simulink library "AEMS_Standard_Library"  (R2016b)
settings: Solver=ode45  StartTime=0.0  StopTime=10.0  RelTol=1e-3
undefined symbols (not defined in the file or in its folder): BkPY, carto, Cbx_extegr, Cbx_lpegrsys, Cbx_portegr, Cnx_bnk_nr_conf, Cnx_cyl_nr_conf, ConfigManagement, configuration_management, Cxx_dcm_io_tmr_end_xxxx, Cxx_dcm_rt_tmr_end, Cxx_DID_xxxx_IO_max, Cxx_DID_xxxx_IO_min, Cxx_egrhsofs, Cxx_vmaniegi, DEM_DEBOUNCE_FREEZE, DEM_DTR_CTL_INVISIBLE, DEM_DTR_CTL_NORMAL, Dem_DtrId2_XXX, Dem_DtrId3_XXX, Dem_DtrId4_XXX, Dem_DtrId5_XXX, Dem_DtrId6_XXX, Dem_DtrId7_XXX, Dem_DtrId8_XXX, Dem_DtrId9_XXX, Dem_DtrId_XXX, Dem_EnableConditionId2_XXX, Dem_EnableConditionId3_XXX, Dem_EnableConditionId4_XXX, Dem_EnableConditionId5_XXX, Dem_EnableConditionId6_XXX, Dem_EnableConditionId7_XXX, Dem_EnableConditionId8_XXX, Dem_EnableConditionId_XXX, Dem_EventId, Dem_EventId2_XXX, Dem_EventId3_XXX, Dem_EventId4_XXX, Dem_EventId5_XXX, Dem_EventId6_XXX, Dem_EventId7_XXX, Dem_EventId8_XXX, Dem_EventId9_XXX, Dem_EventId_Device_Faulttype, Dem_EventId_XXX, DEM_IUMPR_GENERAL_DENOMINATOR, DEM_OPCYC_IGNITION, Dem_RatioId2_XXX, Dem_RatioId3_XXX, Dem_RatioId4_XXX, Dem_RatioId5_XXX, Dem_RatioId6_XXX, Dem_RatioId7_XXX, Dem_RatioId8_XXX, Dem_RatioId_XXX, Dem_StorageConditionId2_XXX, Dem_StorageConditionId3_XXX, Dem_StorageConditionId4_XXX, Dem_StorageConditionId5_XXX ... (+65)
libraries: AEMS_Standard_Library x477, simulink x2
(part 28 of 39)

== system AEMS_Standard_Library/SPECIFIC/AEMS_AT_EHR/A_Enabled_Calculation ==
  Vxx_ehr_sel_tenv : Inport
  Vxx_ehr_cnvt_fac : Inport  Port=2
  Vxx_ehr_ext_exch_ar : Inport  Port=3
  Vxx_ehr_samp_t : Inport  Port=4
  Vxx_ehr_sys_egaf : Inport  Port=5
  Vxx_ehr_wht : Inport  Port=6
  Vxx_ehr_utp : Inport  Port=7
  Vxx_ehr_cata_temp_dly : Inport  Port=8
  Vxx_ehr_exo_pow : Inport  Port=9
  Vxx_ehr_spc_ex_gas_temp_cpy : Inport  Port=10
  Vxx_ehr_spc_cata_temp_cpy : Inport  Port=11
  A_Calcul_for_all_bricks : Subsystem
  B_Temp_calculation_in_brick : Subsystem
  Saturation : Saturate  UpperLimit=65.535  LowerLimit=0  RndMeth=Zero
      settings: AttributesFormatString=<limits=%<UpperLimit>/%<LowerLimit>>
  Vxx_ehr_dtp : Outport
  Vxx_ehr_ext_pow_loss : Outport  Port=2
  Vxx_ehr_wht_entr : Outport  Port=3
  Vxx_ehr_ex_gas_entr : Outport  Port=4
  Vxx_ehr_ext_cnvt_entr : Outport  Port=5
  Vxx_ehr_exo_temp_flu : Outport  Port=6
  Vxx_ehr_wht_temp_flu : Outport  Port=7
  Vxx_ehr_ex_gas_temp_flu : Outport  Port=8
  Vxx_ehr_ext_cnvt_temp_flu : Outport  Port=9
  wires:
  Saturation/1 -> Vxx_ehr_ext_cnvt_entr/1, B_Temp_calculation_in_brick/1(Vxx_ehr_ext_cnvt_entr)
  A_Calcul_for_all_bricks/1(Vxx_ehr_ext_cnvt_entr) -> Saturation/1
  B_Temp_calculation_in_brick/1(Vxx_ehr_dtp) -> Vxx_ehr_dtp/1
  B_Temp_calculation_in_brick/3(Vxx_ehr_wht_entr) -> Vxx_ehr_wht_entr/1
  B_Temp_calculation_in_brick/2(Vxx_ehr_ext_pow_loss) -> Vxx_ehr_ext_pow_loss/1
  Vxx_ehr_sel_tenv/1 -> B_Temp_calculation_in_brick/3(Vxx_ehr_sel_tenv)
  Vxx_ehr_cnvt_fac/1 -> A_Calcul_for_all_bricks/1(Vxx_ehr_cnvt_fac)
  Vxx_ehr_ext_exch_ar/1 -> A_Calcul_for_all_bricks/2(Vxx_ehr_ext_exch_ar)
  Vxx_ehr_samp_t/1 -> A_Calcul_for_all_bricks/3(Vxx_ehr_samp_t), B_Temp_calculation_in_brick/2(Vxx_ehr_samp_t)
  Vxx_ehr_spc_ex_gas_temp_cpy/1 -> B_Temp_calculation_in_brick/4(Vxx_ehr_spc_ex_gas_temp_cpy)
  Vxx_ehr_spc_cata_temp_cpy/1 -> B_Temp_calculation_in_brick/5(Vxx_ehr_spc_cata_temp_cpy)
  Vxx_ehr_sys_egaf/1 -> B_Temp_calculation_in_brick/6(Vxx_ehr_sys_egaf)
  Vxx_ehr_exo_pow/1 -> B_Temp_calculation_in_brick/7(Vxx_ehr_exo_pow)
  Vxx_ehr_wht/1 -> B_Temp_calculation_in_brick/8(Vxx_ehr_wht)
  Vxx_ehr_utp/1 -> B_Temp_calculation_in_brick/9(Vxx_ehr_utp)
  Vxx_ehr_cata_temp_dly/1 -> B_Temp_calculation_in_brick/10(Vxx_ehr_cata_temp_dly)
  B_Temp_calculation_in_brick/8(Vxx_ehr_ext_cnvt_temp_flu) -> Vxx_ehr_ext_cnvt_temp_flu/1
  B_Temp_calculation_in_brick/4(Vxx_ehr_ex_gas_entr) -> Vxx_ehr_ex_gas_entr/1
  B_Temp_calculation_in_brick/5(Vxx_ehr_exo_temp_flu) -> Vxx_ehr_exo_temp_flu/1
  B_Temp_calculation_in_brick/6(Vxx_ehr_wht_temp_flu) -> Vxx_ehr_wht_temp_flu/1
  B_Temp_calculation_in_brick/7(Vxx_ehr_ex_gas_temp_flu) -> Vxx_ehr_ex_gas_temp_flu/1

== system AEMS_Standard_Library/SPECIFIC/AEMS_AT_TUBE/A_Thermal_Calculation ==
  Vxx_tub_utp : Inport
  Vxx_tub_utp_dly : Inport  Port=2
  Vxx_tub_egaf : Inport  Port=3
  Vxx_tub_temp_air : Inport  Port=4
  Vxx_tub_pow_ext : Inport  Port=5
  Vxx_tub_itl_ar : Inport  Port=6
  Vxx_tub_itl_cnvt_fac : Inport  Port=7
  Vxx_tub_ext_ar : Inport  Port=8
  Vxx_tub_ext_cnvt_fac : Inport  Port=9
  Vxx_tub_wht : Inport  Port=10
  Vxx_tub_temp_rd_loss : Inport  Port=11
  Vxx_tub_itl_gas_wht_cor : Inport  Port=12
  Vxx_tub_cal_cpy : Inport  Port=13
  Vxx_tub_gas_cal_cpy : Inport  Port=14
  Vxx_tub_utp_gas_wht_cor : Inport  Port=15
  Vxx_tub_samp_t : Inport  Port=16
  Vxx_tub_temp_esti_dly : Inport  Port=17
  Vxx_tub_ex_gas_dtp_esti_dly : Inport  Port=18
  A_Thermal_Convection_Terms_Tube : Subsystem
  B_Thermal_Material_Model_Tube : Subsystem
  C_Thermal_Gas_Model_Tube : Subsystem
  Saturation : Saturate  UpperLimit=13106  LowerLimit=0  RndMeth=Zero
      settings: AttributesFormatString=<limits=%<UpperLimit>/%<LowerLimit>>
  Saturation1 : Saturate  UpperLimit=65.535  LowerLimit=0  RndMeth=Zero
      settings: AttributesFormatString=<limits=%<UpperLimit>/%<LowerLimit>>
  Saturation2 : Saturate  UpperLimit=32767  LowerLimit=-32767  RndMeth=Zero
      settings: AttributesFormatString=<limits=%<UpperLimit>/%<LowerLimit>>
  Saturation3 : Saturate  UpperLimit=32767  LowerLimit=-32767  RndMeth=Zero
      settings: AttributesFormatString=<limits=%<UpperLimit>/%<LowerLimit>>
  Vxx_tub_ex_gas_dtp_esti : Outport
  Vxx_tub_temp_esti : Outport  Port=2
  Vxx_tub_ex_gas_pow_loss : Outport  Port=3
  Vxx_tub_temp_pow_loss : Outport  Port=4
  Vxx_tub_temp_rd_entr : Outport  Port=5
  Vxx_tub_wht_entr : Outport  Port=6
  Vxx_tub_itl_cnvt_entr : Outport  Port=7
  Vxx_tub_ext_cnvt_entr : Outport  Port=8
  Vxx_tub_entr_tot : Outport  Port=9
  Vxx_tub_ext_cnvt_temp_flu : Outport  Port=10
  Vxx_tub_itl_cnvt_temp_flu : Outport  Port=11
  Vxx_tub_wht_temp_flu : Outport  Port=12
  Vxx_tub_ex_gas_entr : Outport  Port=13
  Vxx_tub_itl_gas_wht_entr : Outport  Port=14
  Vxx_tub_itl_gas_cnvt_entr : Outport  Port=15
  Vxx_tub_gas_entr_tot : Outport  Port=16
  Vxx_tub_gas_temp_flu : Outport  Port=17
  Vxx_tub_gas_wht_temp_flu : Outport  Port=18
  Vxx_tub_gas_itl_cnvt_temp_flu : Outport  Port=19
  Vxx_tub_gas_utp_wht_temp_flu : Outport  Port=20
  Vxx_tub_gas_ext_egy_temp_flu : Outport  Port=21
  wires:
  Saturation3/1 -> Vxx_tub_ex_gas_pow_loss/1
  Saturation2/1 -> Vxx_tub_temp_pow_loss/1
  A_Thermal_Convection_Terms_Tube/1(Vxx_tub_ext_ar_cnvt_fac) -> Saturation1/1
  C_Thermal_Gas_Model_Tube/11(Vxx_tub_gas_ext_egy_temp_flu) -> Vxx_tub_gas_ext_egy_temp_flu/1
  C_Thermal_Gas_Model_Tube/10(Vxx_tub_gas_utp_wht_temp_flu) -> Vxx_tub_gas_utp_wht_temp_flu/1
  C_Thermal_Gas_Model_Tube/9(Vxx_tub_gas_itl_cnvt_temp_flu) -> Vxx_tub_gas_itl_cnvt_temp_flu/1
  C_Thermal_Gas_Model_Tube/8(Vxx_tub_gas_wht_temp_flu) -> Vxx_tub_gas_wht_temp_flu/1
  C_Thermal_Gas_Model_Tube/7(Vxx_tub_gas_temp_flu) -> Vxx_tub_gas_temp_flu/1
  C_Thermal_Gas_Model_Tube/6(Vxx_tub_gas_entr_tot) -> Vxx_tub_gas_entr_tot/1
  C_Thermal_Gas_Model_Tube/5(Vxx_tub_itl_gas_cnvt_entr) -> Vxx_tub_itl_gas_cnvt_entr/1
  C_Thermal_Gas_Model_Tube/4(Vxx_tub_itl_gas_wht_entr) -> Vxx_tub_itl_gas_wht_entr/1
  C_Thermal_Gas_Model_Tube/3(Vxx_tub_ex_gas_entr) -> Vxx_tub_ex_gas_entr/1
  B_Thermal_Material_Model_Tube/10(Vxx_tub_wht_temp_flu) -> Vxx_tub_wht_temp_flu/1
  B_Thermal_Material_Model_Tube/9(Vxx_tub_itl_cnvt_temp_flu) -> Vxx_tub_itl_cnvt_temp_flu/1
  B_Thermal_Material_Model_Tube/8(Vxx_tub_ext_cnvt_temp_flu) -> Vxx_tub_ext_cnvt_temp_flu/1
  B_Thermal_Material_Model_Tube/7(Vxx_tub_entr_tot) -> Vxx_tub_entr_tot/1
  B_Thermal_Material_Model_Tube/6(Vxx_tub_ext_cnvt_entr) -> Vxx_tub_ext_cnvt_entr/1
  B_Thermal_Material_Model_Tube/5(Vxx_tub_itl_cnvt_entr) -> Vxx_tub_itl_cnvt_entr/1
  B_Thermal_Material_Model_Tube/4(Vxx_tub_wht_entr) -> Vxx_tub_wht_entr/1
  B_Thermal_Material_Model_Tube/3(Vxx_tub_temp_rd_entr) -> Vxx_tub_temp_rd_entr/1
  Vxx_tub_utp_dly/1 -> C_Thermal_Gas_Model_Tube/9(Vxx_tub_utp_dly)
  Vxx_tub_samp_t/1 -> B_Thermal_Material_Model_Tube/2(Vxx_tub_samp_t), C_Thermal_Gas_Model_Tube/2(Vxx_tub_samp_t)
  Vxx_tub_ex_gas_dtp_esti_dly/1 -> B_Thermal_Material_Model_Tube/10(Vxx_tub_ex_gas_dtp_esti_dly), C_Thermal_Gas_Model_Tube/11(Vxx_tub_ex_gas_dtp_esti_dly)
  Vxx_tub_temp_esti_dly/1 -> B_Thermal_Material_Model_Tube/9(Vxx_tub_temp_esti_dly), C_Thermal_Gas_Model_Tube/10(Vxx_tub_temp_esti_dly)
  Vxx_tub_utp/1 -> C_Thermal_Gas_Model_Tube/8(Vxx_tub_utp)
  Vxx_tub_utp_gas_wht_cor/1 -> C_Thermal_Gas_Model_Tube/6(Vxx_tub_utp_gas_wht_cor)
  Vxx_tub_itl_cnvt_fac/1 -> A_Thermal_Convection_Terms_Tube/1(Vxx_tub_itl_cnvt_fac)
  Vxx_tub_pow_ext/1 -> C_Thermal_Gas_Model_Tube/4(Vxx_tub_pow_ext)
  Vxx_tub_gas_cal_cpy/1 -> C_Thermal_Gas_Model_Tube/7(Vxx_tub_gas_cal_cpy)
  Vxx_tub_itl_gas_wht_cor/1 -> C_Thermal_Gas_Model_Tube/5(Vxx_tub_itl_gas_wht_cor)
  Vxx_tub_temp_air/1 -> B_Thermal_Material_Model_Tube/8(Vxx_tub_temp_air)
  Vxx_tub_temp_rd_loss/1 -> B_Thermal_Material_Model_Tube/6(Vxx_tub_temp_rd_loss)
  Vxx_tub_cal_cpy/1 -> B_Thermal_Material_Model_Tube/7(Vxx_tub_cal_cpy)
  Vxx_tub_wht/1 -> B_Thermal_Material_Model_Tube/5(Vxx_tub_wht)
  Vxx_tub_ext_ar/1 -> A_Thermal_Convection_Terms_Tube/4(Vxx_tub_ext_ar), B_Thermal_Material_Model_Tube/4(Vxx_tub_ext_ar)
  Vxx_tub_itl_ar/1 -> A_Thermal_Convection_Terms_Tube/2(Vxx_tub_itl_ar)
  Vxx_tub_ext_cnvt_fac/1 -> A_Thermal_Convection_Terms_Tube/3(Vxx_tub_ext_cnvt_fac)
  Vxx_tub_egaf/1 -> C_Thermal_Gas_Model_Tube/3(Vxx_tub_egaf)
  C_Thermal_Gas_Model_Tube/1(Vxx_tub_ex_gas_dtp_esti) -> Vxx_tub_ex_gas_dtp_esti/1
  B_Thermal_Material_Model_Tube/1(Vxx_tub_temp_esti) -> Vxx_tub_temp_esti/1
  A_Thermal_Convection_Terms_Tube/2(Vxx_tub_itl_ar_cnvt_fac) -> Saturation/1
  C_Thermal_Gas_Model_Tube/2(Vxx_tub_ex_gas_pow_loss) -> Saturation3/1
  B_Thermal_Material_Model_Tube/2(Vxx_tub_temp_pow_loss) -> Saturation2/1
  Saturation1/1 -> B_Thermal_Material_Model_Tube/1(Vxx_tub_ext_ar_cnvt_fac)
  Saturation/1 -> B_Thermal_Material_Model_Tube/3(Vxx_tub_itl_ar_cnvt_fac), C_Thermal_Gas_Model_Tube/1(Vxx_tub_itl_ar_cnvt_fac)

== system AEMS_Standard_Library/SPECIFIC/AEMS_DGN_BB_RESULT/DGN_BB_Result_Counter ==
  dataclr : Inport  Interpolate=off
  fdgn_raw : Inport  Port=2  PortDimensions=1  Interpolate=off
  fdgn_fs : Inport  Port=3
  fdgn_nbc : Inport  Port=4
  mdgn_ngt : Inport  Port=5  Interpolate=off
  mdgn_ngc : Inport  Port=6  Interpolate=off
  mdgn_hc : Inport  Port=7  Interpolate=off
  fdgn_avl : Inport  Port=8  PortDimensions=1  Interpolate=off
  fdgn_dgnsw : EnablePort
      settings: AttributesFormatString=<states=%<StatesWhenEnabling>>
  AEMS_SRFLIPFLOP1 : AEMS_Standard_Library/FLAG/AEMS_SRFLIPFLOP  Tag=[LIB]  init=false
      settings: AttributesFormatString=%<MaskType>\nInitial condition (state of Q): = %<init>
  AEMS_SRFLIPFLOP2 : AEMS_Standard_Library/FLAG/AEMS_SRFLIPFLOP  Tag=[LIB]  init=false
      settings: AttributesFormatString=%<MaskType>\nInitial condition (state of Q): = %<init>
  Constant2 : Constant  Value=0  OutDataTypeStr=uint16
  Constant3 : Constant  Value=0  OutDataTypeStr=uint16
  Constant6 : Constant  Value=0  OutDataTypeStr=uint16
  Logical Operator2 : Logic  Operator=OR  Inputs=3  OutDataTypeStr=boolean
  Logical Operator4 : Logic  OutDataTypeStr=boolean
  MinMax3 : MinMax  Function=max  Inputs=2  SaturateOnIntegerOverflow=on  InputSameDT=on
  MinMax5 : MinMax  Inputs=2  SaturateOnIntegerOverflow=on  InputSameDT=on
  MinMax6 : MinMax  Inputs=2  SaturateOnIntegerOverflow=on  InputSameDT=on
  Relational Operator1 : RelationalOperator  Operator=<=  OutDataTypeStr=boolean  RndMeth=Nearest  InputSameDT=on
  Relational Operator2 : RelationalOperator  Operator===  OutDataTypeStr=boolean  RndMeth=Nearest  InputSameDT=on
  Relational Operator3 : RelationalOperator  Operator=<=  OutDataTypeStr=boolean  RndMeth=Nearest  InputSameDT=on
  Sum1 : Sum  Inputs=+-  SaturateOnIntegerOverflow=on  InputSameDT=on
  Sum2 : Sum  Inputs=+-  SaturateOnIntegerOverflow=on  InputSameDT=on
  Sum3 : Sum  SaturateOnIntegerOverflow=on  InputSameDT=on
  Sum4 : Sum  Inputs=+-  SaturateOnIntegerOverflow=on  InputSameDT=on
  Sum5 : Sum  SaturateOnIntegerOverflow=on  InputSameDT=on
  Switch{1..4,7} (5 alike) : Switch  Criteria=u2 ~= 0  SaturateOnIntegerOverflow=on  InputSameDT=on
      settings: AttributesFormatString=Criteria=%<Criteria>
  Unit Delay3 : UnitDelay  SampleTime=-1
      settings: AttributesFormatString=<initial=%<InitialCondition>>
  Unit Delay4 : UnitDelay  SampleTime=-1
      settings: AttributesFormatString=<initial=%<InitialCondition>>
  vdgn_okcnt : Outport  SourceOfInitialOutputValue=Input signal  InitialOutput=0
  vdgn_cnt : Outport  Port=2  SourceOfInitialOutputValue=Input signal  InitialOutput=0
  fdgn_fsok : Outport  Port=3  SourceOfInitialOutputValue=Input signal  InitialOutput=0
  fdgn_dgntrp : Outport  Port=4  SourceOfInitialOutputValue=Input signal  InitialOutput=0
  fdgn_dgnok : Outport  Port=5  SourceOfInitialOutputValue=Input signal  InitialOutput=0
  wires:
  fdgn_fs/1 -> Logical Operator4/2
  Logical Operator4/1 -> fdgn_fsok/1  "fdgn_fsok"
  Switch2/1 -> Switch1/1
  Relational Operator2/1 -> Logical Operator4/1
  Constant2/1 -> Relational Operator2/2
  Unit Delay3/1 -> MinMax3/1, MinMax5/2, Switch1/3  "vdgn_cnt_pudt"
  mdgn_ngt/1 -> Relational Operator3/1, Relational Operator1/1, Sum1/1, Sum2/1
  fdgn_raw/1 -> Switch2/2, Logical Operator2/2
  fdgn_avl/1 -> Switch1/2, Switch4/2
  dataclr/1 -> Logical Operator2/3, Switch3/2, AEMS_SRFLIPFLOP2/2, AEMS_SRFLIPFLOP1/2
  Sum4/1 -> Switch2/3
  Sum3/1 -> Switch2/1
  Switch1/1 -> Switch3/3
  Switch3/1 -> Relational Operator1/2, Unit Delay3/1, Relational Operator2/1, vdgn_cnt/1  "vdgn_cnt"
  Constant3/1 -> Switch3/1
  Unit Delay4/1 -> MinMax6/2, Switch4/3  "vgpfrmvp_cnt_pudt"
  Switch4/1 -> Switch7/3
  Switch7/1 -> Relational Operator3/2, Unit Delay4/1, vdgn_okcnt/1  "vdgn_okcnt"
  Constant6/1 -> Switch7/1
  Logical Operator2/1 -> Switch7/2
  fdgn_nbc/1 -> Logical Operator2/1
  mdgn_ngc/1 -> Sum5/1, Sum2/2, Sum3/1, Sum1/2
  MinMax3/1 -> Sum4/1
  mdgn_hc/1 -> Sum4/2, MinMax3/2
  Sum2/1 -> MinMax5/1
  MinMax5/1 -> Sum3/2
  Sum1/1 -> MinMax6/1
  MinMax6/1 -> Sum5/2
  Sum5/1 -> Switch4/1
  Relational Operator3/1 -> AEMS_SRFLIPFLOP1/1  "set"
  Relational Operator1/1 -> AEMS_SRFLIPFLOP2/1  "set"
  AEMS_SRFLIPFLOP1/1 -> fdgn_dgnok/1  "fdgn_dgnok"
  AEMS_SRFLIPFLOP2/1 -> fdgn_dgntrp/1  "fdgn_dgntrp"

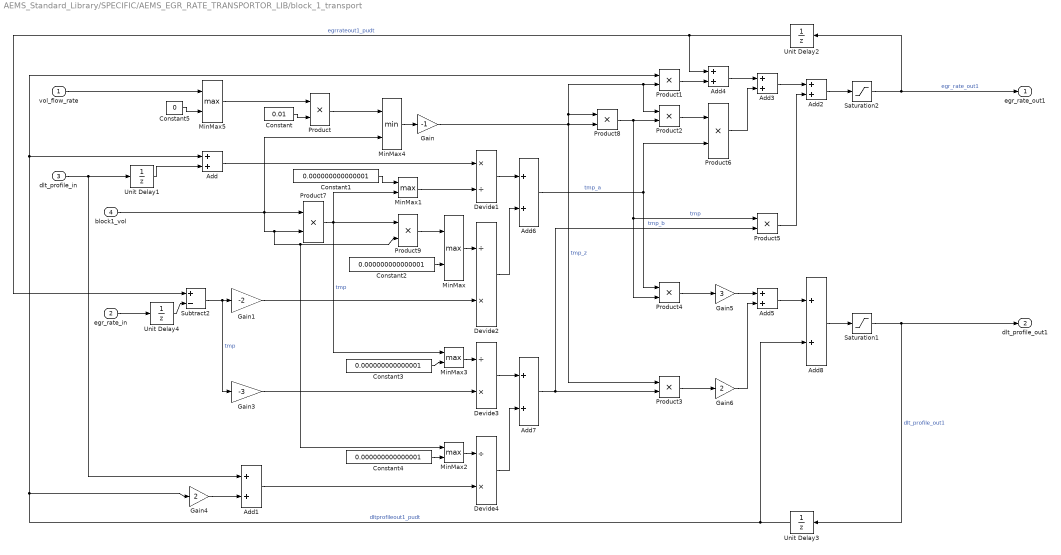
== system AEMS_Standard_Library/SPECIFIC/AEMS_EGR_RATE_TRANSPORTOR_LIB/block_1_transport ==
  vol_flow_rate : Inport
  egr_rate_in : Inport  Port=2
  dlt_profile_in : Inport  Port=3
  block1_vol : Inport  Port=4
  Add{,1..8} (9 alike) : Sum  SaturateOnIntegerOverflow=on  InputSameDT=on
  Constant : Constant  Value=0.01  OutDataTypeStr=single
  Constant{1..4} (4 alike) : Constant  Value=0.000000000000001  OutDataTypeStr=single
  Constant5 : Constant  Value=0  OutDataTypeStr=single
  Devide1 : Product  Inputs=*/  OutDataTypeStr=Inherit: Inherit via back propagation
  Devide2 : Product  Inputs=/*  OutDataTypeStr=Inherit: Inherit via back propagation
  Devide3 : Product  Inputs=/*  OutDataTypeStr=Inherit: Inherit via back propagation
  Devide4 : Product  Inputs=/*  OutDataTypeStr=Inherit: Inherit via back propagation
  Gain : Gain  Gain=-1  ParamDataTypeStr=single  SaturateOnIntegerOverflow=on
  Gain1 : Gain  Gain=-2  ParamDataTypeStr=single  SaturateOnIntegerOverflow=on
  Gain3 : Gain  Gain=-3  ParamDataTypeStr=single  SaturateOnIntegerOverflow=on
  Gain4 : Gain  Gain=2  ParamDataTypeStr=single  SaturateOnIntegerOverflow=on
  Gain5 : Gain  Gain=3  ParamDataTypeStr=single  SaturateOnIntegerOverflow=on
  Gain6 : Gain  Gain=2  ParamDataTypeStr=single  SaturateOnIntegerOverflow=on
  MinMax{,1..3,5} (5 alike) : MinMax  Function=max  Inputs=2  SaturateOnIntegerOverflow=on  InputSameDT=on
  MinMax4 : MinMax  Inputs=2  SaturateOnIntegerOverflow=on  InputSameDT=on
  Product{,1..9} (10 alike) : Product  OutDataTypeStr=Inherit: Inherit via back propagation  RndMeth=Zero
  Saturation1 : Saturate  UpperLimit=1000  LowerLimit=-1000
      settings: AttributesFormatString=<limits=%<UpperLimit>/%<LowerLimit>>
  Saturation2 : Saturate  UpperLimit=1  LowerLimit=0
      settings: AttributesFormatString=<limits=%<UpperLimit>/%<LowerLimit>>
  Subtract2 : Sum  Inputs=+-  SaturateOnIntegerOverflow=on  InputSameDT=on
  Unit Delay{1..4} (4 alike) : UnitDelay  SampleTime=-1
      settings: AttributesFormatString=<initial=%<InitialCondition>>
  egr_rate_out1 : Outport
  dlt_profile_out1 : Outport  Port=2
  wires:
  MinMax4/1 -> Gain/1
  Product/1 -> MinMax4/1
  Gain/1 -> Product1/2, Product2/1, Product8/1, Product3/1, Product8/2  "tmp_z"
  Constant/1 -> Product/2
  Constant3/1 -> MinMax3/2
  Constant4/1 -> MinMax2/2
  MinMax1/1 -> Devide1/2
  Constant1/1 -> MinMax1/1
  Add2/1 -> Saturation2/1
  vol_flow_rate/1 -> MinMax5/1
  Add8/1 -> Saturation1/1
  Add5/1 -> Add8/1
  Gain6/1 -> Add5/2
  Gain5/1 -> Add5/1
  Product3/1 -> Gain6/1
  Product4/1 -> Gain5/1
  Product5/1 -> Add2/2
  Add3/1 -> Add2/1
  Product6/1 -> Add3/2
  Add4/1 -> Add3/1
  Product1/1 -> Add4/2
  Product8/1 -> Product4/2, Product5/1, Product2/2  "tmp"
  Add7/1 -> Product3/2, Product5/2  "tmp_b"
  Add6/1 -> Product4/1, Product6/2  "tmp_a"
  Product2/1 -> Product6/1
  Gain4/1 -> Add1/2
  Add/1 -> Devide1/1
  block1_vol/1 -> Product7/1, MinMax4/2, MinMax2/1, Product9/2, Product7/2
  Product7/1 -> MinMax3/1, MinMax1/2, Product9/1  "tmp"
  Subtract2/1 -> Gain3/1, Gain1/1  "tmp"
  dlt_profile_in/1 -> Add1/1, Unit Delay1/1
  egr_rate_in/1 -> Unit Delay4/1
  Unit Delay2/1 -> Subtract2/1, Add4/1  "egrrateout1_pudt"
  Unit Delay3/1 -> Gain4/1, Add/1, Product1/1, Add8/2  "dltprofileout1_pudt"
  Devide1/1 -> Add6/1
  Devide2/1 -> Add6/2
  Product9/1 -> MinMax/1
  Constant2/1 -> MinMax/2
  MinMax/1 -> Devide2/1
  Gain1/1 -> Devide2/2
  Add1/1 -> Devide4/2
  MinMax2/1 -> Devide4/1
  MinMax3/1 -> Devide3/1
  Gain3/1 -> Devide3/2
  Devide3/1 -> Add7/1
  Devide4/1 -> Add7/2
  Constant5/1 -> MinMax5/2
  MinMax5/1 -> Product/1
  Saturation2/1 -> egr_rate_out1/1, Unit Delay2/1  "egr_rate_out1"
  Saturation1/1 -> Unit Delay3/1, dlt_profile_out1/1  "dlt_profile_out1"
  Unit Delay1/1 -> Add/2
  Unit Delay4/1 -> Subtract2/2

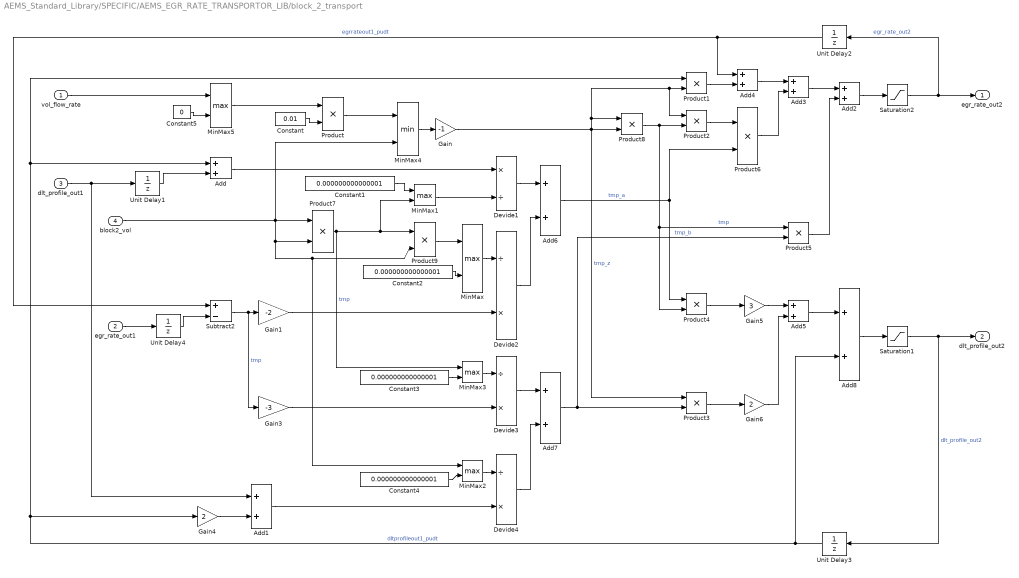
== system AEMS_Standard_Library/SPECIFIC/AEMS_EGR_RATE_TRANSPORTOR_LIB/block_2_transport ==
  vol_flow_rate : Inport
  egr_rate_out1 : Inport  Port=2
  dlt_profile_out1 : Inport  Port=3
  block2_vol : Inport  Port=4
  Add{,1..8} (9 alike) : Sum  SaturateOnIntegerOverflow=on  InputSameDT=on
  Constant : Constant  Value=0.01  OutDataTypeStr=single
  Constant{1..4} (4 alike) : Constant  Value=0.000000000000001  OutDataTypeStr=single
  Constant5 : Constant  Value=0  OutDataTypeStr=single
  Devide1 : Product  Inputs=*/  OutDataTypeStr=Inherit: Inherit via back propagation
  Devide2 : Product  Inputs=/*  OutDataTypeStr=Inherit: Inherit via back propagation
  Devide3 : Product  Inputs=/*  OutDataTypeStr=Inherit: Inherit via back propagation
  Devide4 : Product  Inputs=/*  OutDataTypeStr=Inherit: Inherit via back propagation
  Gain : Gain  Gain=-1  ParamDataTypeStr=single  SaturateOnIntegerOverflow=on
  Gain1 : Gain  Gain=-2  ParamDataTypeStr=single  SaturateOnIntegerOverflow=on
  Gain3 : Gain  Gain=-3  ParamDataTypeStr=single  SaturateOnIntegerOverflow=on
  Gain4 : Gain  Gain=2  ParamDataTypeStr=single  SaturateOnIntegerOverflow=on
  Gain5 : Gain  Gain=3  ParamDataTypeStr=single  SaturateOnIntegerOverflow=on
  Gain6 : Gain  Gain=2  ParamDataTypeStr=single  SaturateOnIntegerOverflow=on
  MinMax{,1..3,5} (5 alike) : MinMax  Function=max  Inputs=2  SaturateOnIntegerOverflow=on  InputSameDT=on
  MinMax4 : MinMax  Inputs=2  SaturateOnIntegerOverflow=on  InputSameDT=on
  Product{,1..9} (10 alike) : Product  OutDataTypeStr=Inherit: Inherit via back propagation  RndMeth=Zero
  Saturation1 : Saturate  UpperLimit=1000  LowerLimit=-1000
      settings: AttributesFormatString=<limits=%<UpperLimit>/%<LowerLimit>>
  Saturation2 : Saturate  UpperLimit=1  LowerLimit=0
      settings: AttributesFormatString=<limits=%<UpperLimit>/%<LowerLimit>>
  Subtract2 : Sum  Inputs=+-  SaturateOnIntegerOverflow=on  InputSameDT=on
  Unit Delay{1..4} (4 alike) : UnitDelay  SampleTime=-1
      settings: AttributesFormatString=<initial=%<InitialCondition>>
  egr_rate_out2 : Outport
  dlt_profile_out2 : Outport  Port=2
  wires:
  Saturation1/1 -> dlt_profile_out2/1, Unit Delay3/1  "dlt_profile_out2"
  Saturation2/1 -> Unit Delay2/1, egr_rate_out2/1  "egr_rate_out2"
  MinMax5/1 -> Product/1
  Constant5/1 -> MinMax5/2
  Devide4/1 -> Add7/2
  Devide3/1 -> Add7/1
  Gain3/1 -> Devide3/2
  MinMax3/1 -> Devide3/1
  MinMax2/1 -> Devide4/1
  Add1/1 -> Devide4/2
  Gain1/1 -> Devide2/2
  MinMax/1 -> Devide2/1
  Constant2/1 -> MinMax/2
  Product9/1 -> MinMax/1
  Devide2/1 -> Add6/2
  Devide1/1 -> Add6/1
  Unit Delay3/1 -> Gain4/1, Add/1, Product1/1, Add8/2  "dltprofileout1_pudt"
  Unit Delay2/1 -> Add4/1, Subtract2/1  "egrrateout1_pudt"
  egr_rate_out1/1 -> Unit Delay4/1
  dlt_profile_out1/1 -> Add1/1, Unit Delay1/1
  Subtract2/1 -> Gain1/1, Gain3/1  "tmp"
  Product7/1 -> MinMax3/1, MinMax1/2, Product9/1  "tmp"
  block2_vol/1 -> MinMax4/2, Product7/1, MinMax2/1, Product9/2, Product7/2
  Add/1 -> Devide1/1
  Gain4/1 -> Add1/2
  Product2/1 -> Product6/1
  Add6/1 -> Product6/2, Product4/1  "tmp_a"
  Add7/1 -> Product3/2, Product5/2  "tmp_b"
  Product8/1 -> Product2/2, Product5/1, Product4/2  "tmp"
  Product1/1 -> Add4/2
  Add4/1 -> Add3/1
  Product6/1 -> Add3/2
  Add3/1 -> Add2/1
  Product5/1 -> Add2/2
  Product4/1 -> Gain5/1
  Product3/1 -> Gain6/1
  Gain5/1 -> Add5/1
  Gain6/1 -> Add5/2
  Add5/1 -> Add8/1
  Add8/1 -> Saturation1/1
  vol_flow_rate/1 -> MinMax5/1
  Add2/1 -> Saturation2/1
  Constant1/1 -> MinMax1/1
  MinMax1/1 -> Devide1/2
  Constant4/1 -> MinMax2/2
  Constant3/1 -> MinMax3/2
  Constant/1 -> Product/2
  Gain/1 -> Product8/2, Product3/1, Product8/1, Product2/1, Product1/2  "tmp_z"
  Product/1 -> MinMax4/1
  MinMax4/1 -> Gain/1
  Unit Delay1/1 -> Add/2
  Unit Delay4/1 -> Subtract2/2

== system AEMS_Standard_Library/SPECIFIC/AEMS_EGR_RATE_TRANSPORTOR_LIB/block_3_transport ==
  vol_flow_rate : Inport
  egr_rate_out2 : Inport  Port=2
  dlt_profile_out2 : Inport  Port=3
  block3_vol : Inport  Port=4
  Add{,1..8} (9 alike) : Sum  SaturateOnIntegerOverflow=on  InputSameDT=on
  Constant : Constant  Value=0.01  OutDataTypeStr=single
  Constant{1..4} (4 alike) : Constant  Value=0.000000000000001  OutDataTypeStr=single
  Constant5 : Constant  Value=0  OutDataTypeStr=single
  Devide1 : Product  Inputs=*/  OutDataTypeStr=Inherit: Inherit via back propagation
  Devide2 : Product  Inputs=/*  OutDataTypeStr=Inherit: Inherit via back propagation
  Devide3 : Product  Inputs=/*  OutDataTypeStr=Inherit: Inherit via back propagation
  Devide4 : Product  Inputs=/*  OutDataTypeStr=Inherit: Inherit via back propagation
  Gain : Gain  Gain=-1  ParamDataTypeStr=single  SaturateOnIntegerOverflow=on
  Gain1 : Gain  Gain=-2  ParamDataTypeStr=single  SaturateOnIntegerOverflow=on
  Gain3 : Gain  Gain=-3  ParamDataTypeStr=single  SaturateOnIntegerOverflow=on
  Gain4 : Gain  Gain=2  ParamDataTypeStr=single  SaturateOnIntegerOverflow=on
  Gain5 : Gain  Gain=3  ParamDataTypeStr=single  SaturateOnIntegerOverflow=on
  Gain6 : Gain  Gain=2  ParamDataTypeStr=single  SaturateOnIntegerOverflow=on
  MinMax{,1..3,5} (5 alike) : MinMax  Function=max  Inputs=2  SaturateOnIntegerOverflow=on  InputSameDT=on
  MinMax4 : MinMax  Inputs=2  SaturateOnIntegerOverflow=on  InputSameDT=on
  Product{,1..9} (10 alike) : Product  OutDataTypeStr=Inherit: Inherit via back propagation  RndMeth=Zero
  Saturation1 : Saturate  UpperLimit=1000  LowerLimit=-1000
      settings: AttributesFormatString=<limits=%<UpperLimit>/%<LowerLimit>>
  Saturation2 : Saturate  UpperLimit=1  LowerLimit=0
      settings: AttributesFormatString=<limits=%<UpperLimit>/%<LowerLimit>>
  Subtract2 : Sum  Inputs=+-  SaturateOnIntegerOverflow=on  InputSameDT=on
  Unit Delay{1..4} (4 alike) : UnitDelay  SampleTime=-1
      settings: AttributesFormatString=<initial=%<InitialCondition>>
  egr_rate_out3 : Outport
  dlt_profile_out3 : Outport  Port=2
  wires:
  Add/1 -> Devide1/1
  block3_vol/1 -> Product7/1, Product7/2, MinMax2/1, Product9/2, MinMax4/2
  MinMax4/1 -> Gain/1
  Product/1 -> MinMax4/1
  Gain/1 -> Product1/2, Product2/1, Product8/1, Product3/1, Product8/2  "tmp_z"
  Constant/1 -> Product/2
  Constant3/1 -> MinMax3/2
  Constant4/1 -> MinMax2/2
  MinMax1/1 -> Devide1/2
  Constant1/1 -> MinMax1/1
  Add2/1 -> Saturation2/1
  vol_flow_rate/1 -> MinMax5/1
  Add8/1 -> Saturation1/1
  Add5/1 -> Add8/1
  Gain6/1 -> Add5/2
  Gain5/1 -> Add5/1
  Product3/1 -> Gain6/1
  Product4/1 -> Gain5/1
  Product5/1 -> Add2/2
  Add3/1 -> Add2/1
  Product6/1 -> Add3/2
  Add4/1 -> Add3/1
  Product1/1 -> Add4/2
  Product8/1 -> Product4/2, Product5/1, Product2/2  "tmp"
  Add7/1 -> Product3/2, Product5/2  "tmp_b"
  Add6/1 -> Product4/1, Product6/2  "tmp_a"
  Product2/1 -> Product6/1
  Gain4/1 -> Add1/2
  Product7/1 -> MinMax1/2, Product9/1, MinMax3/1  "tmp"
  Subtract2/1 -> Gain3/1, Gain1/1  "tmp"
  dlt_profile_out2/1 -> Add1/1, Unit Delay1/1
  egr_rate_out2/1 -> Unit Delay4/1
  Unit Delay2/1 -> Subtract2/1, Add4/1  "egrrateout1_pudt"
  Unit Delay3/1 -> Gain4/1, Add/1, Product1/1, Add8/2  "dltprofileout1_pudt"
  Devide1/1 -> Add6/1
  Devide2/1 -> Add6/2
  Product9/1 -> MinMax/1
  Constant2/1 -> MinMax/2
  MinMax/1 -> Devide2/1
  Gain1/1 -> Devide2/2
  Add1/1 -> Devide4/2
  MinMax2/1 -> Devide4/1
  MinMax3/1 -> Devide3/1
  Gain3/1 -> Devide3/2
  Devide3/1 -> Add7/1
  Devide4/1 -> Add7/2
  Constant5/1 -> MinMax5/2
  MinMax5/1 -> Product/1
  Saturation2/1 -> egr_rate_out3/1, Unit Delay2/1  "egr_rate_out3"
  Saturation1/1 -> Unit Delay3/1, dlt_profile_out3/1  "dlt_profile_out3"
  Unit Delay1/1 -> Add/2
  Unit Delay4/1 -> Subtract2/2

== system AEMS_Standard_Library/SPECIFIC/AEMS_EGR_RATE_TRANSPORTOR_LIB/dlt_profile_output_selector ==
  dlt_profile_out3 : Inport
  dlt_profile_out2 : Inport  Port=2
  dlt_profile_out1 : Inport  Port=3
  block_selector : Inport  Port=4
  Multiport Switch : MultiPortSwitch  SaturateOnIntegerOverflow=on  InputSameDT=on
  Saturation2 : Saturate  UpperLimit=3  LowerLimit=1
      settings: AttributesFormatString=<limits=%<UpperLimit>/%<LowerLimit>>
  dlt_profile_out : Outport
  wires:
  Multiport Switch/1 -> dlt_profile_out/1  "dlt_profile_out"
  dlt_profile_out3/1 -> Multiport Switch/4
  dlt_profile_out2/1 -> Multiport Switch/3
  dlt_profile_out1/1 -> Multiport Switch/2
  block_selector/1 -> Saturation2/1
  Saturation2/1 -> Multiport Switch/1

== system AEMS_Standard_Library/SPECIFIC/AEMS_EGR_RATE_TRANSPORTOR_LIB/egr_rate_output_selector ==
  block_selector : Inport
  egr_rate_out1 : Inport  Port=2
  egr_rate_out2 : Inport  Port=3
  egr_rate_out3 : Inport  Port=4
  Multiport Switch : MultiPortSwitch  SaturateOnIntegerOverflow=on  InputSameDT=on
  Saturation2 : Saturate  UpperLimit=3  LowerLimit=1
      settings: AttributesFormatString=<limits=%<UpperLimit>/%<LowerLimit>>
  egr_rate_out : Outport
  wires:
  block_selector/1 -> Saturation2/1
  egr_rate_out1/1 -> Multiport Switch/2
  egr_rate_out2/1 -> Multiport Switch/3
  egr_rate_out3/1 -> Multiport Switch/4
  Multiport Switch/1 -> egr_rate_out/1  "egr_rate_out"
  Saturation2/1 -> Multiport Switch/1

== system AEMS_Standard_Library/SPECIFIC/AEMS_MULTIPORT_TIMESWITCH_CONFIG/Get_input_and_input_old ==
  Select_Input_old : Inport
  Select_Input : Inport  Port=2
  Inputs : Inport  Port=3
  Selector : Selector  InputPortWidth=LimitDimInputs  IndexOptions=Index vector (port)  Indices=[1 3]  OutputSizes=1
  Selector1 : Selector  InputPortWidth=LimitDimInputs  IndexOptions=Index vector (port)  Indices=[1 3]  OutputSizes=1
  Vxx_in : Outport
  Vxx_in_old : Outport  Port=2
  wires:
  Select_Input_old/1 -> Selector1/2
  Inputs/1 -> Selector/1, Selector1/1
  Select_Input/1 -> Selector/2
  Selector1/1 -> Vxx_in_old/1
  Selector/1 -> Vxx_in/1

== system AEMS_Standard_Library/SPECIFIC/AEMS_MULTIPORT_TIMESWITCH_CONFIG/in_clc ==
  Vnx_swi_nr_stt : Inport
  Vbx_sel_puls : Inport  Port=2
  Vxx_in : Inport  Port=3
  Vxx_in_old : Inport  Port=4
  Constant1 : Constant  Value=2  OutDataTypeStr=Inherit: Inherit via back propagation
  Constant3 : Constant  OutDataTypeStr=Inherit: Inherit via back propagation
  Relational_Operator11 : RelationalOperator  Operator===  OutDataTypeStr=boolean  RndMeth=Nearest  InputSameDT=on
  Relational_Operator41 : RelationalOperator  Operator===  OutDataTypeStr=boolean  RndMeth=Nearest  InputSameDT=on
  Switch : Switch  Criteria=u2 ~= 0  RndMeth=Zero  SaturateOnIntegerOverflow=on  InputSameDT=on
      settings: AttributesFormatString=Criteria=%<Criteria>
  Switch1 : Switch  Criteria=u2 ~= 0  RndMeth=Zero  SaturateOnIntegerOverflow=on  InputSameDT=on
      settings: AttributesFormatString=Criteria=%<Criteria>
  Switch2 : Switch  Criteria=u2 ~= 0  RndMeth=Zero  SaturateOnIntegerOverflow=on  InputSameDT=on
      settings: AttributesFormatString=Criteria=%<Criteria>
  Unit_Delay11 : UnitDelay  SampleTime=-1
      settings: AttributesFormatString=<initial=%<InitialCondition>>
  Unit_Delay3 : UnitDelay  SampleTime=-1
      settings: AttributesFormatString=<initial=%<InitialCondition>>
  Vxx_out_sel : Outport
  Vxx_out_sel_old : Outport  Port=2
  wires:
  Vbx_sel_puls/1 -> Switch1/2
  Relational_Operator11/1 -> Switch2/2
  Constant1/1 -> Relational_Operator11/2
  Relational_Operator41/1 -> Switch/2
  Constant3/1 -> Relational_Operator41/2
  Vxx_in_old/1 -> Switch2/1
  Unit_Delay11/1 -> Switch2/3
  Switch2/1 -> Unit_Delay11/1, Switch1/3
  Switch1/1 -> Vxx_out_sel_old/1
  Vxx_in/1 -> Switch/1
  Vnx_swi_nr_stt/1 -> Relational_Operator41/1, Relational_Operator11/1
  Unit_Delay3/1 -> Switch1/1, Switch/3
  Switch/1 -> Unit_Delay3/1, Vxx_out_sel/1

== system AEMS_Standard_Library/SPECIFIC/AEMS_MULTIPORT_TIMESWITCH_CONFIG/interpolation ==
  Vxx_out_sel : Inport
  Vxx_out_sel_old : Inport  Port=2
  Slop_on : Inport  Port=3
  Vxx_swi_trs : Inport  Port=4
  AEMS_CLAMP : AEMS_Standard_Library/MATH/AEMS_CLAMP  Tag=[LIB]
      settings: AttributesFormatString=%<MaskType>
  Constant11 : Constant  OutDataTypeStr=Inherit: Inherit via back propagation
  MinMax : MinMax  Inputs=2  OutDataTypeStr=Inherit: Inherit via back propagation  RndMeth=Zero  InputSameDT=on
  MinMax1 : MinMax  Function=max  Inputs=2  OutDataTypeStr=Inherit: Inherit via back propagation  RndMeth=Zero  InputSameDT=on
  Product1 : Product  Inputs=**  OutDataTypeStr=Inherit: Inherit via back propagation  RndMeth=Zero
  Product2 : Product  Inputs=**  OutDataTypeStr=Inherit: Inherit via back propagation  RndMeth=Zero
  Sum2 : Sum  Inputs=+-  OutDataTypeStr=Inherit: Inherit via back propagation  RndMeth=Zero  InputSameDT=on
  Sum5 : Sum  OutDataTypeStr=Inherit: Inherit via back propagation  RndMeth=Zero  InputSameDT=on
  Switch : Switch  Criteria=u2 ~= 0  RndMeth=Zero  SaturateOnIntegerOverflow=on  InputSameDT=on
      settings: AttributesFormatString=Criteria=%<Criteria>
  Output : Outport
  wires:
  MinMax/1 -> AEMS_CLAMP/3
  MinMax1/1 -> AEMS_CLAMP/1
  AEMS_CLAMP/1 -> Output/1
  Vxx_out_sel/1 -> MinMax/1, Switch/3, Product1/2, MinMax1/1
  Vxx_out_sel_old/1 -> Product2/1, MinMax1/2, MinMax/2
  Product1/1 -> Sum5/2
  Vxx_swi_trs/1 -> Product1/1, Sum2/2
  Constant11/1 -> Sum2/1
  Switch/1 -> AEMS_CLAMP/2
  Slop_on/1 -> Switch/2
  Product2/1 -> Sum5/1
  Sum5/1 -> Switch/1
  Sum2/1 -> Product2/2

== system AEMS_Standard_Library/SPECIFIC/AEMS_MULTIPORT_TIMESWITCH_CONFIG/number_1_2 ==
  Slop_on : Inport
  Vbx_sel_puls : Inport  Port=2
  Constant1 : Constant  OutDataTypeStr=uint8
  Constant11 : Constant  OutDataTypeStr=Inherit: Inherit via back propagation
  Constant2 : Constant  Value=2  OutDataTypeStr=Inherit: Inherit via back propagation
  Logical_Operator : Logic  Operator=OR  OutDataTypeStr=boolean
  Logical_Operator1 : Logic  OutDataTypeStr=boolean
  Logical_Operator2 : Logic  Operator=NOT  Inputs=1  OutDataTypeStr=boolean
  Relational_Operator : RelationalOperator  OutDataTypeStr=boolean  RndMeth=Nearest  InputSameDT=on
  Sum2 : Sum  OutDataTypeStr=Inherit: Inherit via back propagation  RndMeth=Zero  SaturateOnIntegerOverflow=on  InputSameDT=on
      settings: AttributesFormatString=SAT = %<SaturateOnIntegerOverflow>
  Switch : Switch  Criteria=u2 ~= 0  RndMeth=Zero  SaturateOnIntegerOverflow=on  InputSameDT=on
      settings: AttributesFormatString=Criteria=%<Criteria>
  Unit_Delay2 : UnitDelay  InitialCondition=1  SampleTime=-1
      settings: AttributesFormatString=<initial=%<InitialCondition>>
  Vnx_swi_nr_stt : Outport
  wires:
  Logical_Operator/1 -> Logical_Operator2/1
  Logical_Operator2/1 -> Logical_Operator1/1
  Constant2/1 -> Relational_Operator/2
  Relational_Operator/1 -> Logical_Operator/1
  Constant1/1 -> Switch/3
  Sum2/1 -> Switch/1
  Unit_Delay2/1 -> Relational_Operator/1, Sum2/1
  Constant11/1 -> Sum2/2
  Switch/1 -> Unit_Delay2/1, Vnx_swi_nr_stt/1
  Logical_Operator1/1 -> Switch/2
  Vbx_sel_puls/1 -> Logical_Operator/2
  Slop_on/1 -> Logical_Operator1/2

== system AEMS_Standard_Library/SPECIFIC/AEMS_MULTIPORT_TIMESWITCH_CONFIG/pulse_and_old ==
  Select_Input : Inport
  AEMS_UNITDELAY_EXTERNALIC : AEMS_Standard_Library/DISCRETE/AEMS_UNITDELAY_EXTERNALIC  Tag=[LIB]
      settings: AttributesFormatString=%<MaskType>
  Relational_Operator : RelationalOperator  Operator=~=  OutDataTypeStr=boolean  RndMeth=Nearest  InputSameDT=on
  Switch : Switch  Criteria=u2 ~= 0  RndMeth=Zero  SaturateOnIntegerOverflow=on  InputSameDT=on
      settings: AttributesFormatString=Criteria=%<Criteria>
  Unit_Delay : UnitDelay  InitialCondition=1  SampleTime=-1
      settings: AttributesFormatString=<initial=%<InitialCondition>>
  Vbx_sel_puls : Outport
  Select_Input_old : Outport  Port=2
  wires:
  Unit_Delay/1 -> Switch/3
  Switch/1 -> Unit_Delay/1, Select_Input_old/1
  Relational_Operator/1 -> Switch/2, Vbx_sel_puls/1
  Select_Input/1 -> Relational_Operator/2, AEMS_UNITDELAY_EXTERNALIC/2, AEMS_UNITDELAY_EXTERNALIC/1
  AEMS_UNITDELAY_EXTERNALIC/1 -> Relational_Operator/1, Switch/1

== system AEMS_Standard_Library/SPECIFIC/AEMS_MULTIPORT_TIMESWITCH_CONFIG/slop_on ==
  Vxx_swi_trs : Inport
  Vbx_sel_puls : Inport  Port=2
  Constant3 : Constant  OutDataTypeStr=Inherit: Inherit via back propagation
  Relational_Operator4 : RelationalOperator  OutDataTypeStr=boolean  RndMeth=Nearest  InputSameDT=on
  SR_FlipFlop : Subsystem  mask(SRFlipFlop){initial_condition=0}
      mask prompts: initial_condition "Initial condition:"
      mask help: S-R Flip Flop Block
  Terminator : Terminator
  Slop_on : Outport
  wires:
  SR_FlipFlop/2(QNot) -> Terminator/1
  SR_FlipFlop/1(Q) -> Slop_on/1
  Vxx_swi_trs/1 -> Relational_Operator4/1
  Vbx_sel_puls/1 -> SR_FlipFlop/1(S)
  Constant3/1 -> Relational_Operator4/2
  Relational_Operator4/1 -> SR_FlipFlop/2(R)

== system AEMS_Standard_Library/SPECIFIC/AEMS_MULTIPORT_TIMESWITCH_CONFIG/transient_timer ==
  Duration : Inport
  dT : Inport  Port=2
  Vbx_sel_puls : Inport  Port=3
  Constant{1..2,4..5} (4 alike) : Constant  OutDataTypeStr=Inherit: Inherit via back propagation
  Constant3 : Constant  Value=0  OutDataTypeStr=Inherit: Inherit via back propagation
  DivisionByZero : Subsystem
  FixPt_Unit_Delay2 : UnitDelay  DisableCoverage=on  SampleTime=-1
      settings: AttributesFormatString=<initial=%<InitialCondition>>
  LogicalOperator : Logic  Operator=OR  OutDataTypeStr=boolean
  Relational_Operator1 : RelationalOperator  OutDataTypeStr=boolean  RndMeth=Nearest  InputSameDT=on
  Relational_Operator2 : RelationalOperator  Operator=>  OutDataTypeStr=boolean  RndMeth=Nearest  InputSameDT=on
  Relational_Operator3 : RelationalOperator  OutDataTypeStr=boolean  RndMeth=Nearest  InputSameDT=on
  Sum : Sum  OutDataTypeStr=Inherit: Inherit via back propagation  RndMeth=Zero  InputSameDT=on
  Sum1 : Sum  OutDataTypeStr=Inherit: Inherit via back propagation  RndMeth=Zero  InputSameDT=on
  Switch{,1..3} (4 alike) : Switch  Criteria=u2 ~= 0  RndMeth=Zero  SaturateOnIntegerOverflow=on  InputSameDT=on
      settings: AttributesFormatString=Criteria=%<Criteria>
  UnitDelayResettable : Subsystem
  Vxx_swi_trs : Outport
  wires:
  Relational_Operator2/1 -> LogicalOperator/1
  LogicalOperator/1 -> Switch3/2
  DivisionByZero/1(ans) -> Switch3/1, Relational_Operator2/1
  Relational_Operator1/1 -> Switch2/2
  Constant5/1 -> Relational_Operator1/2
  Vbx_sel_puls/1 -> UnitDelayResettable/2(R), LogicalOperator/2, Switch/2
  Duration/1 -> Sum1/1
  FixPt_Unit_Delay2/1 -> Relational_Operator1/1, Switch3/3, Relational_Operator2/2
  Relational_Operator3/1 -> Switch1/2
  Constant3/1 -> Switch2/1
  Switch2/1 -> Sum/1
  dT/1 -> Switch2/3, Switch/1
  Sum/1 -> DivisionByZero/2(num), Switch/3
  UnitDelayResettable/1(y) -> Sum/2
  Switch/1 -> Sum1/2, UnitDelayResettable/1(u)
  Sum1/1 -> DivisionByZero/1(den)
  Switch3/1 -> FixPt_Unit_Delay2/1, Switch1/3, Relational_Operator3/1
  Switch1/1 -> Vxx_swi_trs/1
  Constant1/1 -> Relational_Operator3/2
  Constant2/1 -> Switch1/1
  Constant4/1 -> DivisionByZero/3(ans_of_0div)

== system AEMS_Standard_Library/SPECIFIC/AEMS_SlopeSwitchExtern/Estimate_transition_time ==
  note: Current Input
  note: Current Output
  note: Avoid A Division by Zero
  Input : Inport
  Output : Inport  Port=2
  Pos_Slope : Inport  Port=3
  Neg_Slope : Inport  Port=4
  Constant1 : Constant  Value=-1  OutDataTypeStr=Inherit: Inherit via back propagation
  Constant3 : Constant  Value=1.1921e-07  OutDataTypeStr=Inherit: Inherit via back propagation
  Divide2 : Product  Inputs=*/  OutDataTypeStr=Inherit: Inherit via back propagation  RndMeth=Zero
  MinMax3 : MinMax  Function=max  Inputs=2  OutDataTypeStr=Inherit: Inherit via back propagation  RndMeth=Zero  InputSameDT=on
  Product : Product  OutDataTypeStr=Inherit: Inherit via back propagation  RndMeth=Zero
  RelationalOperator : RelationalOperator  Operator=>  OutDataTypeStr=boolean  RndMeth=Nearest  InputSameDT=on
  Subtract1 : Sum  Inputs=+-  OutDataTypeStr=Inherit: Inherit via back propagation  RndMeth=Zero  InputSameDT=on
  Subtract2 : Sum  Inputs=+-  OutDataTypeStr=Inherit: Inherit via back propagation  RndMeth=Zero  InputSameDT=on
  Switch1 : Switch  Criteria=u2 ~= 0  RndMeth=Zero  InputSameDT=on
      settings: AttributesFormatString=Criteria=%<Criteria>
  Switch2 : Switch  Criteria=u2 ~= 0  RndMeth=Zero  InputSameDT=on
      settings: AttributesFormatString=Criteria=%<Criteria>
  Rem_Transition_Time : Outport
  wires:
  Subtract1/1 -> Switch2/3
  Switch2/1 -> Divide2/1
  Divide2/1 -> Rem_Transition_Time/1
  Input/1 -> Subtract2/1, Subtract1/2, RelationalOperator/1
  Output/1 -> Subtract2/2, Subtract1/1, RelationalOperator/2
  RelationalOperator/1 -> Switch2/2, Switch1/2
  Constant1/1 -> Product/2
  Product/1 -> Switch1/3
  Neg_Slope/1 -> Product/1
  Subtract2/1 -> Switch2/1
  Pos_Slope/1 -> Switch1/1
  Constant3/1 -> MinMax3/2
  Switch1/1 -> MinMax3/1
  MinMax3/1 -> Divide2/2

== system AEMS_Standard_Library/SPECIFIC/AEMS_SlopeSwitchExtern/Signal_Change_Compute ==
  Switch_Cmd : Inport
  Relational_Operator : RelationalOperator  Operator=~=  OutDataTypeStr=boolean  RndMeth=Nearest  InputSameDT=on
  UnitDelay : UnitDelay  SampleTime=-1
      settings: AttributesFormatString=<initial=%<InitialCondition>>
  Signal_Change : Outport
  wires:
  Switch_Cmd/1 -> UnitDelay/1, Relational_Operator/1
  Relational_Operator/1 -> Signal_Change/1
  UnitDelay/1 -> Relational_Operator/2

== system AEMS_Standard_Library/SPECIFIC/AEMS_SlopeSwitchExtern/Slope_On_Block ==
  Signal_Change : Inport
  Input : Inport  Port=2
  Pos_Slope : Inport  Port=3
  Neg_Slope : Inport  Port=4
  Prev_Output : Inport  Port=5
  Slope_On : EnablePort
      settings: AttributesFormatString=StatesWhenEnabling: %<StatesWhenEnabling>
  Error_Due_To_High_Slope_Test : Subsystem
  Output_Comparision : Subsystem
  Output_Not_Equals_Input : Outport
      settings: AttributesFormatString=<initial=%<InitialOutput>>\n<whendisabled=%<OutputWhenDisabled>>
  Output : Outport  Port=2
      settings: AttributesFormatString=<initial=%<InitialOutput>>\n<whendisabled=%<OutputWhenDisabled>>
  wires:
  Output_Comparision/4(Output_Greater_Than_Input) -> Error_Due_To_High_Slope_Test/3(Output_Greater_Than_Input)
  Output_Comparision/3(Output_Less_Than_Input) -> Error_Due_To_High_Slope_Test/2(Output_Less_Than_Input)
  Neg_Slope/1 -> Output_Comparision/5(Neg_Slope)
  Input/1 -> Output_Comparision/2(Input)
  Pos_Slope/1 -> Output_Comparision/3(Pos_Slope)
  Prev_Output/1 -> Output_Comparision/4(Prev_Output)
  Error_Due_To_High_Slope_Test/1(Test_passed) -> Output_Comparision/1(Test_passed)
  Output_Comparision/2(Output) -> Output/1
  Output_Comparision/1(Output_Not_Equals_Input) -> Output_Not_Equals_Input/1
  Signal_Change/1 -> Error_Due_To_High_Slope_Test/1(Signal_Change)

== system AEMS_Standard_Library/SPECIFIC/AEMS_SlopeSwitchExtern/Slope_On_Compute ==
  Signal_Change : Inport
  Output_Not_Equals_Input : Inport  Port=2
  Constant1 : Constant  Value=false
  Constant3 : Constant  Value=true
  LogicalOperator : Logic  Operator=OR  OutDataTypeStr=boolean
  Switch2 : Switch  Criteria=u2 ~= 0  RndMeth=Zero  SaturateOnIntegerOverflow=on  InputSameDT=on
      settings: AttributesFormatString=Criteria=%<Criteria>
  UnitDelay1 : UnitDelay  InitialCondition=false  SampleTime=-1
      settings: AttributesFormatString=<initial=%<InitialCondition>>
  Slope_On : Outport
  wires:
  Switch2/1 -> LogicalOperator/2
  Constant1/1 -> Switch2/3
  Constant3/1 -> UnitDelay1/1
  UnitDelay1/1 -> Switch2/2
  Signal_Change/1 -> Switch2/1
  LogicalOperator/1 -> Slope_On/1
  Output_Not_Equals_Input/1 -> LogicalOperator/1

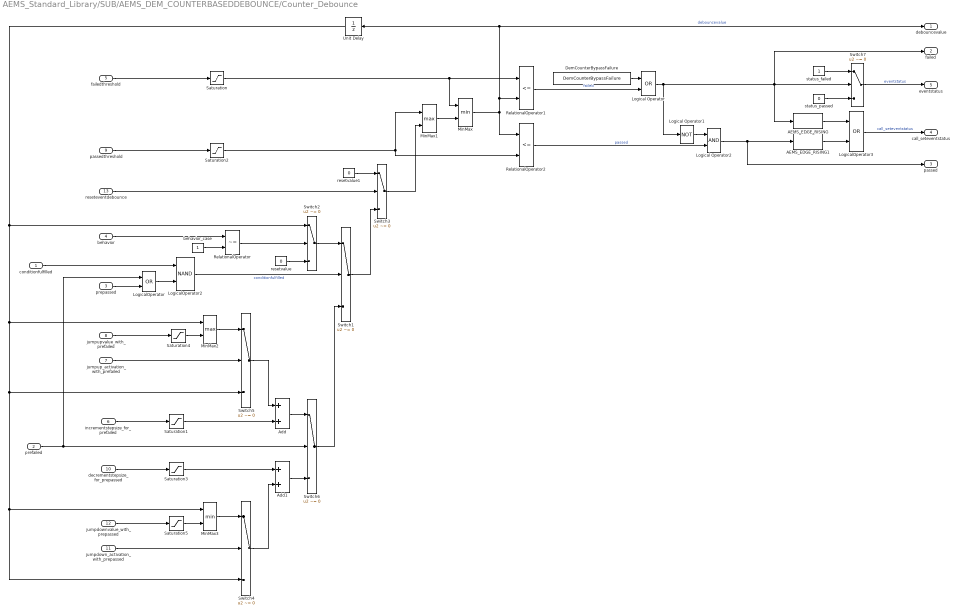
== system AEMS_Standard_Library/SUB/AEMS_DEM_COUNTERBASEDDEBOUNCE/Counter_Debounce ==
  conditionfulfilled : Inport
  prefailed : Inport  Port=2
  prepassed : Inport  Port=3
  behavior : Inport  Port=4
  failedthreshold : Inport  Port=5
  incrementstepsize_for_prefailed : Inport  Port=6
  jumpup_activation_with_prefailed : Inport  Port=7
  jumpupvalue_with_prefailed : Inport  Port=8
  passedthreshold : Inport  Port=9
  decrementstepsize_for_prepassed : Inport  Port=10
  jumpdown_activation_with_prepassed : Inport  Port=11
  jumpdownvalue_with_prepassed : Inport  Port=12
  reseteventdebounce : Inport  Port=13
  AEMS_EDGE_RISING : AEMS_Standard_Library/EDGE/AEMS_EDGE_RISING  Tag=[LIB]  init=false
      settings: AttributesFormatString=|
      | %<MaskType>
      | Initial Value : %<init>
  AEMS_EDGE_RISING1 : AEMS_Standard_Library/EDGE/AEMS_EDGE_RISING  Tag=[LIB]  init=false
      settings: AttributesFormatString=|
      | %<MaskType>
      | Initial Value : %<init>
  Add : Sum  OutDataTypeStr=Inherit: Inherit via back propagation  SaturateOnIntegerOverflow=on  InputSameDT=on
      settings: AttributesFormatString=SAT = %<SaturateOnIntegerOverflow>
  Add1 : Sum  OutDataTypeStr=Inherit: Inherit via back propagation  SaturateOnIntegerOverflow=on  InputSameDT=on
      settings: AttributesFormatString=SAT = %<SaturateOnIntegerOverflow>
  DemCounterBypassFailure : Constant  Value=DemCounterBypassFailure
  Logical Operator : Logic  Operator=OR  OutDataTypeStr=boolean
  Logical Operator1 : Logic  Operator=NOT  OutDataTypeStr=boolean
  Logical Operator2 : Logic  OutDataTypeStr=boolean
  LogicalOperator : Logic  Operator=OR  OutDataTypeStr=boolean
  LogicalOperator2 : Logic  Operator=NAND  OutDataTypeStr=boolean
  LogicalOperator3 : Logic  Operator=OR  OutDataTypeStr=boolean
  MinMax : MinMax  Inputs=2  InputSameDT=on
  MinMax1 : MinMax  Function=max  Inputs=2  OutDataTypeStr=Inherit: Inherit via back propagation  InputSameDT=on
  MinMax2 : MinMax  Function=max  Inputs=2  InputSameDT=on
  MinMax3 : MinMax  Inputs=2  InputSameDT=on
  RelationalOperator : RelationalOperator  Operator=~=  OutDataTypeStr=boolean  RndMeth=Nearest  InputSameDT=on
  RelationalOperator1 : RelationalOperator  Operator=<=  OutDataTypeStr=boolean  RndMeth=Nearest  InputSameDT=on
  RelationalOperator2 : RelationalOperator  Operator=<=  OutDataTypeStr=boolean  RndMeth=Nearest  InputSameDT=on
  Saturation : Saturate  UpperLimit=32767  LowerLimit=1
      settings: AttributesFormatString=<limits=%<UpperLimit>/%<LowerLimit>>
  Saturation1 : Saturate  UpperLimit=32767  LowerLimit=1
      settings: AttributesFormatString=<limits=%<UpperLimit>/%<LowerLimit>>
  Saturation2 : Saturate  UpperLimit=-1  LowerLimit=-32768
      settings: AttributesFormatString=<limits=%<UpperLimit>/%<LowerLimit>>
  Saturation3 : Saturate  UpperLimit=-1  LowerLimit=-32768
      settings: AttributesFormatString=<limits=%<UpperLimit>/%<LowerLimit>>
  Saturation4 : Saturate  UpperLimit=32767  LowerLimit=-32768
      settings: AttributesFormatString=<limits=%<UpperLimit>/%<LowerLimit>>
  Saturation5 : Saturate  UpperLimit=32767  LowerLimit=-32768
      settings: AttributesFormatString=<limits=%<UpperLimit>/%<LowerLimit>>
  Switch{1..7} (7 alike) : Switch  Criteria=u2 ~= 0  SaturateOnIntegerOverflow=on  InputSameDT=on
      settings: AttributesFormatString=Criteria=%<Criteria>
  Unit Delay : UnitDelay  SampleTime=-1
      settings: AttributesFormatString=<initial=%<InitialCondition>>
  behavior_case : Constant  OutDataTypeStr=uint8
  resetvalue : Constant  Value=0  OutDataTypeStr=int16
  resetvalue1 : Constant  Value=0  OutDataTypeStr=int16
  status_failed : Constant  OutDataTypeStr=uint8
  status_passed : Constant  Value=0  OutDataTypeStr=uint8
  debouncevalue : Outport
  failed : Outport  Port=2
  passed : Outport  Port=3
  call_seteventstatus : Outport  Port=4
  eventstatus : Outport  Port=5
  wires:
  Logical Operator1/1 -> Logical Operator2/1
  Logical Operator2/1 -> passed/1, AEMS_EDGE_RISING1/1
  conditionfulfilled/1 -> LogicalOperator2/1
  LogicalOperator2/1 -> Switch1/2  "conditionfulfilled"
  MinMax3/1 -> Switch4/1
  MinMax2/1 -> Switch5/1
  prepassed/1 -> LogicalOperator/2
  Unit Delay/1 -> Switch2/1, MinMax2/1, Switch4/3, MinMax3/1, Switch5/3
  LogicalOperator3/1 -> call_seteventstatus/1  "call_seteventstatus"
  AEMS_EDGE_RISING1/1 -> LogicalOperator3/2
  AEMS_EDGE_RISING/1 -> LogicalOperator3/1
  RelationalOperator2/1 -> Logical Operator2/2  "passed"
  Switch7/1 -> eventstatus/1  "eventstatus"
  status_passed/1 -> Switch7/3
  status_failed/1 -> Switch7/1
  MinMax/1 -> Unit Delay/1, debouncevalue/1, RelationalOperator1/2, RelationalOperator2/1  "debouncevalue"
  MinMax1/1 -> MinMax/2
  Saturation2/1 -> RelationalOperator2/2, MinMax1/1
  Saturation/1 -> RelationalOperator1/1, MinMax/1
  Switch6/1 -> Switch1/3
  Add1/1 -> Switch6/3
  Add/1 -> Switch6/1
  Saturation3/1 -> Add1/1
  Switch4/1 -> Add1/2
  Saturation1/1 -> Add/2
  Switch5/1 -> Add/1
  Saturation4/1 -> MinMax2/2
  resetvalue1/1 -> Switch3/1
  Switch3/1 -> MinMax1/2
  reseteventdebounce/1 -> Switch3/2
  RelationalOperator/1 -> Switch2/2
  behavior_case/1 -> RelationalOperator/2
  Switch1/1 -> Switch3/3
  resetvalue/1 -> Switch2/3
  Switch2/1 -> Switch1/1
  Saturation5/1 -> MinMax3/2
  jumpdownvalue_with_prepassed/1 -> Saturation5/1
  jumpdown_activation_with_prepassed/1 -> Switch4/2
  decrementstepsize_for_prepassed/1 -> Saturation3/1
  passedthreshold/1 -> Saturation2/1
  jumpupvalue_with_prefailed/1 -> Saturation4/1
  jumpup_activation_with_prefailed/1 -> Switch5/2
  incrementstepsize_for_prefailed/1 -> Saturation1/1
  prefailed/1 -> LogicalOperator/1, Switch6/2
  LogicalOperator/1 -> LogicalOperator2/2
  failedthreshold/1 -> Saturation/1
  behavior/1 -> RelationalOperator/1
  DemCounterBypassFailure/1 -> Logical Operator/1
  Logical Operator/1 -> Logical Operator1/1, failed/1, Switch7/2, AEMS_EDGE_RISING/1
  RelationalOperator1/1 -> Logical Operator/2  "failed"

== system AEMS_Standard_Library/SUB/AEMS_DEM_COUNTERBASEDDEBOUNCE/Dem_SetEventStatus_Call ==
  event_status : Inport
  call_seteventstatus : EnablePort
      settings: AttributesFormatString=<states=%<StatesWhenEnabling>>
  AEMS_DEM_SETEVENTSTATUS : AEMS_Standard_Library/SUB/AEMS_DEM_SETEVENTSTATUS  Tag=[LIB]
      settings: AttributesFormatString=%<MaskType>
  EventId_block : Constant  Value=Dem_EventId_Device_Faulttype  OutDataTypeStr=uint16
  wires:
  event_status/1 -> AEMS_DEM_SETEVENTSTATUS/2
  EventId_block/1 -> AEMS_DEM_SETEVENTSTATUS/1
